simulink model "SG8_MPC_simu_MPC_student"  (R2020b)
settings: Solver=VariableStepAuto  StartTime=0.0  StopTime=40  RelTol=1e-3
undefined symbols (not defined in the file): A, A_OBS, Amaxpred, Arefpred, B, B_OBS, Bmaxpred, Brefpred, C, C_OBS, Cmaxpred, Crefpred, D, D_OBS, Dmaxpred, Drefpred, F, H, lambda_e, lambda_u, Np, sigbuilder_block, Te
settings Model: Creator=rbourdais  LastModifiedBy=ouyang

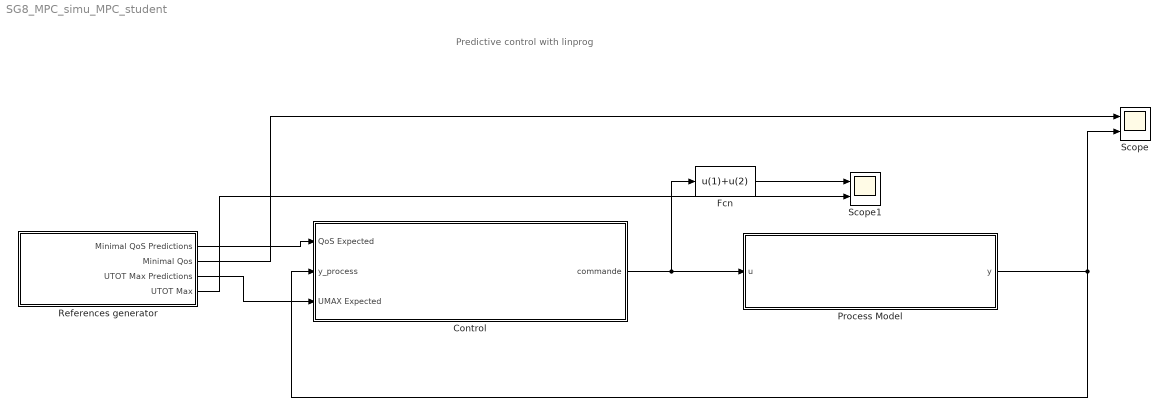
== system SG8_MPC_simu_MPC_student ==
  note: Predictive control with linprog
  Control : Subsystem
  Fcn : Fcn  Expr=u(1)+u(2)
  Process Model : Subsystem
  References generator : Subsystem
  Scope : Scope  NumInputPorts=2
  Scope1 : Scope  NumInputPorts=2
  wires:
  References generator/1(Minimal QoS Predictions) -> Control/1(QoS Expected)
  Control/1(commande) -> Fcn/1, Process Model/1(u)
  Process Model/1(y) -> Scope/2, Control/2(y_process)
  References generator/2(Minimal Qos) -> Scope/1
  References generator/3(UTOT Max Predictions) -> Control/3(UMAX Expected)
  References generator/4(UTOT Max) -> Scope1/2
  Fcn/1 -> Scope1/1

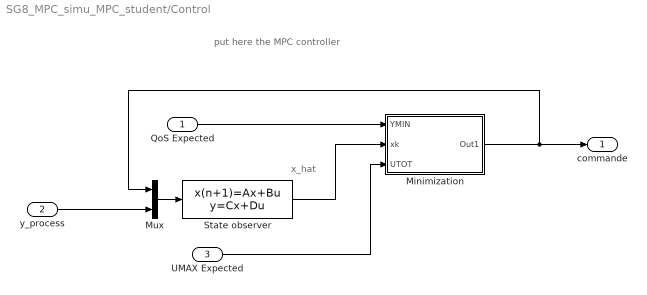
== system SG8_MPC_simu_MPC_student/Control ==
  note: x_hat
  note: put here the MPC controller
  QoS Expected : Inport
  y_process : Inport  Port=2
  UMAX Expected : Inport  Port=3
  Minimization : Subsystem
  Mux : Mux  Inputs=2
  State observer : DiscreteStateSpace  A=A_OBS  B=B_OBS  C=C_OBS  D=D_OBS  SampleTime=Te
  commande : Outport
  wires:
  y_process/1 -> Mux/2
  Mux/1 -> State observer/1
  Minimization/1(Out1) -> commande/1, Mux/1
  QoS Expected/1 -> Minimization/1(YMIN)
  State observer/1 -> Minimization/2(xk)
  UMAX Expected/1 -> Minimization/3(UTOT)

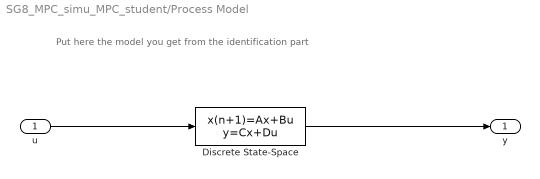
== system SG8_MPC_simu_MPC_student/Process Model ==
  note: Put here the model you get from the identification part
  u : Inport
  Discrete State-Space : DiscreteStateSpace  A=A  B=B  C=C  D=D  SampleTime=Te
  y : Outport
  wires:
  u/1 -> Discrete State-Space/1
  Discrete State-Space/1 -> y/1

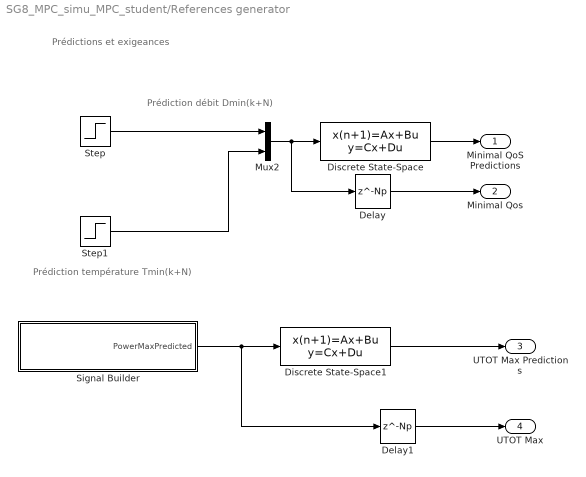
== system SG8_MPC_simu_MPC_student/References generator ==
  note: Prédiction débit Dmin(k+N)
  note: Prédictions et exigeances
  note: Prédiction température Tmin(k+N)
  Delay : Delay  DelayLength=Np  SampleTime=Te
  Delay1 : Delay  DelayLength=Np  InitialCondition=15  SampleTime=Te
  Discrete State-Space : DiscreteStateSpace  A=Arefpred  B=Brefpred  C=Crefpred  D=Drefpred  SampleTime=Te
  Discrete State-Space1 : DiscreteStateSpace  A=Amaxpred  B=Bmaxpred  C=Cmaxpred  D=Dmaxpred  InitialCondition=15*ones(Np,1)  SampleTime=Te
  Mux2 : Mux  Inputs=2
  Signal Builder : Subsystem  Tag=STV Subsys  LoadFcn=sigbuilder_block('load');  StartFcn=sigbuilder_block('start');  StopFcn=sigbuilder_block('stop');  ClipboardFcn=sigbuilder_block('clipboard');  mask(Sigbuilder block){tuvar=[0:10]}
      mask help: Simulink:masks:SigbuilderBlock_MD
      mask init:
      | if ~strcmp(get_param(bdroot(gcbh),'SimulationStatus'),'stopped') tuvar = sigbuilder_block('maskInit'); end
      settings: CopyFcn=sigbuilder_block('copy');  DeleteFcn=sigbuilder_block('delete');  ModelCloseFcn=sigbuilder_block('modelClose');  PreSaveFcn=sigbuilder_block('preSave');  PauseFcn=sigbuilder_block('pause');  ContinueFcn=sigbuilder_block('continue');  NameChangeFcn=sigbuilder_block('namechange');  OpenFcn=sigbuilder_block('open',[147.75 264 550.5 359.25 ]);  CloseFcn=sigbuilder_block('close');
      mask Display: plot(0, 0, 100, 100,[2, 2, 32, 32, 2], [68, 8, 8, 68, 68],[32, 2], [38, 38], [32, 19, 2],[53, 60, 44], [32, 17, 17, 2],[16, 16, 31, 31]);txt = getActiveGroup(gcbh);text(2, 100, txt,'verticalAlignment', 'top');
  Step : Step  Time=3  Before=5  After=5.5  SampleTime=0
  Step1 : Step  Time=7  Before=3  After=3  SampleTime=0
  Minimal QoS Predictions : Outport
  Minimal Qos : Outport  Port=2
  UTOT Max Predictions : Outport  Port=3
  UTOT Max : Outport  Port=4
  wires:
  Step/1 -> Mux2/1
  Step1/1 -> Mux2/2
  Mux2/1 -> Delay/1, Discrete State-Space/1
  Discrete State-Space/1 -> Minimal QoS Predictions/1
  Delay/1 -> Minimal Qos/1
  Signal Builder/1(PowerMaxPredicted) -> Delay1/1, Discrete State-Space1/1
  Discrete State-Space1/1 -> UTOT Max Predictions/1
  Delay1/1 -> UTOT Max/1

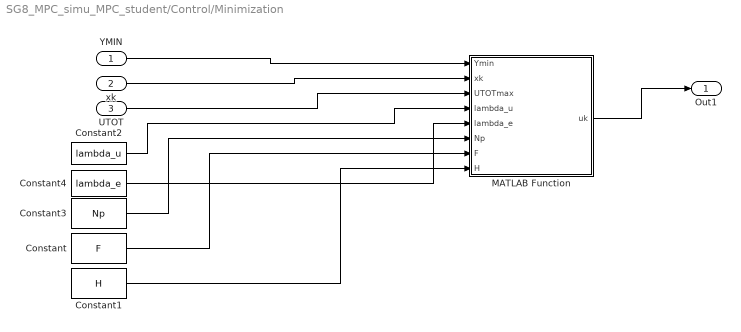
== system SG8_MPC_simu_MPC_student/Control/Minimization ==
  YMIN : Inport
  xk : Inport  Port=2
  UTOT : Inport  Port=3
  Constant : Constant  Value=F
  Constant1 : Constant  Value=H
  Constant2 : Constant  Value=lambda_u
  Constant3 : Constant  Value=Np
  Constant4 : Constant  Value=lambda_e
  MATLAB Function : MATLAB Function  TreatAsAtomicUnit=on
  Out1 : Outport
  wires:
  xk/1 -> MATLAB Function/2(xk)
  YMIN/1 -> MATLAB Function/1(Ymin)
  MATLAB Function/1(uk) -> Out1/1
  UTOT/1 -> MATLAB Function/3(UTOTmax)
  Constant/1 -> MATLAB Function/7(F)
  Constant1/1 -> MATLAB Function/8(H)
  Constant3/1 -> MATLAB Function/6(Np)
  Constant2/1 -> MATLAB Function/4(lambda_u)
  Constant4/1 -> MATLAB Function/5(lambda_e)

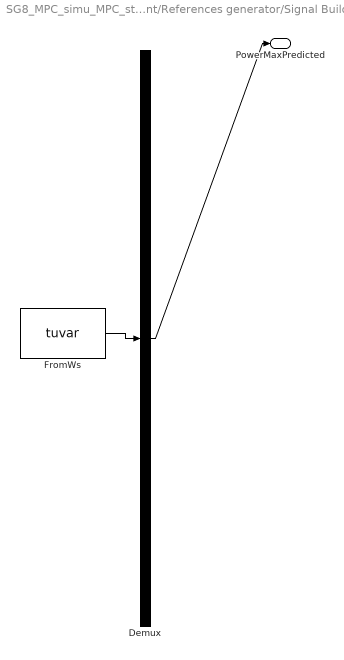
== system SG8_MPC_simu_MPC_student/References generator/Signal Builder ==
  Demux : Demux  Tag=STV Demux  Outputs=1
      settings: DisplayOption=none
  FromWs : FromWorkspace  Tag=STV FromWs  VariableName=tuvar
      SigBuilderData=|
      | common.afterFinalStr = 'Extrapolate'
      | common.sampleTime = 0
      | dataSet.timeRange = [0 20]
      | dataSet.name = 'Group 1'
      | sbobj.Groups.Name = 'Group 1'
      | sbobj.Groups.Signals.Name = 'PowerMaxPredicted'
      | sbobj.Groups.Signals.XData = [0 4 4 5.5 5.5 9 9 10.5 10.5 15 15 16 16 20]
      | sbobj.Groups.Signals.YData = [15 15 8 8 15 15 8 8 15 15 10 10 15 15]
      | sbobj.Groups.TimeRange = [0 20]
  PowerMaxPredicted : Outport  Tag=STV Outport
  wires:
  FromWs/1 -> Demux/1
  Demux/1 -> PowerMaxPredicted/1

== matlab function SG8_MPC_simu_MPC_student/Control/Minimization/MATLAB Function ==
  data: Ymin input; uk output; xk input; UTOTmax input; lambda_u input; lambda_e input; Np input; F input; H input
function uk = fcn(Ymin,xk,UTOTmax,lambda_u,lambda_e, Np, F,H)

uk = [0;0];
coder.extrinsic('quadprog');

% define H and f in quadprog
W = [eye(2*Np), zeros(2*Np,5*Np); zeros(2*Np), lambda_u*eye(2*Np), zeros(2*Np,3*Np); zeros(3*Np,4*Np), lambda_e*eye(3*Np)];
f = [-Ymin', zeros(1,5*Np)];

% define A in quadprog
T = zeros(Np,2*Np);
for i = 1:Np
    T(i,2*i-1:2*i) = [1,1];
end

P = zeros(Np,2*Np);
for i = 1:Np
    P(i,2*i) = 1;
end

Q = zeros(2*Np,3*Np);
for i = 1:Np
    Q(2*i-1,3*i-2) = 1;
    Q(2*i,3*i-1) = 1;
end

R = zeros(Np,3*Np);
for i = 1:Np
    R(i,3*i) = 1;
end

lb = -inf(7*Np,1);
ub = inf(7*Np,1);
lb(2*Np+1:4*Np,1) = 0;
ub(2*Np+1:4*Np,1) = 10;

A = [zeros(Np,2*Np), T, zeros(Np,3*Np); -eye(2*Np), zeros(2*Np), -Q; P, zeros(Np,2*Np), -R];
b = [UTOTmax; -Ymin; P*Ymin + 2*ones(Np,1)];

% Aeq and beq in quadprog 
Aeq = [eye(2*Np), -H, zeros(2*Np,3*Np)];
beq = F*xk;

[Uopt] = quadprog(W,f,A,b,Aeq,beq,lb,ub);

uk = Uopt(2*Np+1:2*Np+2,1)
uk_tot = uk(1)+uk(2)
